simulink model "muscleLegs_task1"  (R2025b)
settings: Solver=ode23t  StartTime=0.0  StopTime=t_end  MaxStep=1e-3  RelTol=1e-4
values from neighbouring files (symbols this model uses):
  c = 0.05    [setup_muscleLegs_nm.m]
  CtrlPar = [tau_H_st; phi_K_tgt_st; P_K_st; D_K_st ... (first row only)    [setup_muscleLegs_ctrl.m]
  eref_se = 0.04    [setup_muscleLegs_nm.m]
  FmaxBFSH = 350    [setup_muscleLegs_nm.m]
  FmaxGLU = 4000    [setup_muscleLegs_nm.m]
  FmaxHFL = 2000    [setup_muscleLegs_nm.m]
  FmaxVAS = 5000    [setup_muscleLegs_nm.m]
  g = 9.81    [setup_muscleLegs_model.m]
  init_stim = 0.01    [setup_muscleLegs_nm.m]
  K = 5    [setup_muscleLegs_nm.m]
  l_shank = l_leg/2    (= 0.49)    [setup_muscleLegs_model.m]
  l_thigh = l_leg/2    (= 0.49)    [setup_muscleLegs_model.m]
  loptBFSH = 0.12    [setup_muscleLegs_nm.m]
  loptGLU = 0.11    [setup_muscleLegs_nm.m]
  loptHFL = 0.11    [setup_muscleLegs_nm.m]
  loptVAS = 0.08    [setup_muscleLegs_nm.m]
  lslackBFSH = 0.10    (= 0.1)    [setup_muscleLegs_nm.m]
  lslackGLU = 0.13    [setup_muscleLegs_nm.m]
  lslackHFL = 0.10    (= 0.1)    [setup_muscleLegs_nm.m]
  lslackVAS = 0.23    [setup_muscleLegs_nm.m]
  m_body = m_total - 2*m_foot    (= 78)    [setup_muscleLegs_model.m]
  m_shank = 4    [setup_muscleLegs_model.m]
  m_thigh = 8    [setup_muscleLegs_model.m]
  N = 12    [cmaes_task1_2_set1.mat]    (also in cmaes_task1_2_set2.mat; cmaes_task2_2_set1.mat = 17; cmaes_task2_2_set2.mat = 17; cmaes_task3_crouch.mat = 17)
  phirefBFSH = 160*pi/180    (= 2.79252680319)    [setup_muscleLegs_nm.m]
  phirefGLU = 60*pi/180    (= 1.0471975512)    [setup_muscleLegs_nm.m]
  phirefHFL = 20*pi/180    (= 0.349065850399)    [setup_muscleLegs_nm.m]
  phirefVAS = 60*pi/180    (= 1.0471975512)    [setup_muscleLegs_nm.m]
  plane_height = 0.1    [setup_muscleLegs_model.m]
  plane_x = 100    [setup_muscleLegs_model.m]
  plane_z = 1    [setup_muscleLegs_model.m]
  r_foot = 0.01    [setup_muscleLegs_model.m]
  rBFSH = 0.04    [setup_muscleLegs_nm.m]
  rGLU = 0.08    [setup_muscleLegs_nm.m]
  rHFL = 0.08    [setup_muscleLegs_nm.m]
  rhoBFSH = 0.7    [setup_muscleLegs_nm.m]
  rhoGLU = 0.5    [setup_muscleLegs_nm.m]
  rhoHFL = 0.5    [setup_muscleLegs_nm.m]
  rhoVAS = 0.6    [setup_muscleLegs_nm.m]
  rVAS = 0.05    [setup_muscleLegs_nm.m]
  tau_act = 0.01    [setup_muscleLegs_nm.m]
  tau_deact = 0.04    [setup_muscleLegs_nm.m]
  vi_Ctrl_st = 1:4    [setup_muscleLegs_ctrl.m]
  vi_Ctrl_sw = 5:12    [setup_muscleLegs_ctrl.m]
  vmaxBFSH = 12    [setup_muscleLegs_nm.m]
  vmaxGLU = 12    [setup_muscleLegs_nm.m]
  vmaxHFL = 12    [setup_muscleLegs_nm.m]
  vmaxVAS = 12    [setup_muscleLegs_nm.m]
  w = 0.56    [setup_muscleLegs_nm.m]
  w_pe = w    (= 0.56)    [setup_muscleLegs_nm.m]
undefined symbols (not defined in the file or in its folder): l1, X, Y, Z
libraries: sm_lib x30, nesl_utility x17, simulink x1
(part 4 of 4)

== system muscleLegs_task1/Muscle Dynamics/MTU7/CE inverse force-velocity relation ==
  note: CE Inverse Force-Velocity Relationship
  Fv[Fmax] : Inport
  1 : Product  Inputs=/*
  Constant{1,3..4,8} (4 alike) : Constant
  Constant2 : Constant  Value=N
  Constant5 : Constant  Value=N
  Curvature : Gain  Gain=K  SaturateOnIntegerOverflow=on  OutDataTypeStr=Inherit: Same as input  ParamDataTypeStr=Inherit: Same as input
  Curvature1 : Gain  Gain=7.56*K  SaturateOnIntegerOverflow=on  OutDataTypeStr=Inherit: Same as input  ParamDataTypeStr=Inherit: Same as input
  Mux : Mux  Inputs=2
  Mux1 : Mux  Inputs=3
  Mux2 : Mux  Inputs=3
  Slope : Gain  Gain=1e-2  SaturateOnIntegerOverflow=on  OutDataTypeStr=Inherit: Same as input  ParamDataTypeStr=Inherit: Same as input
  Sum1 : Sum  Inputs=|++  InputSameDT=on  SaturateOnIntegerOverflow=on  OutDataTypeStr=Inherit: Same as first input
  Sum2 : Sum  InputSameDT=on  SaturateOnIntegerOverflow=on  OutDataTypeStr=Inherit: Same as first input
  Sum3 : Sum  Inputs=++|  InputSameDT=on  SaturateOnIntegerOverflow=on  OutDataTypeStr=Inherit: Same as first input
  Sum4 : Sum  Inputs=|+-  InputSameDT=on  SaturateOnIntegerOverflow=on  OutDataTypeStr=Inherit: Same as first input
  Sum5 : Sum  Inputs=|-+  InputSameDT=on  SaturateOnIntegerOverflow=on  OutDataTypeStr=Inherit: Same as first input
  Sum6 : Sum  Inputs=-+|  InputSameDT=on  SaturateOnIntegerOverflow=on  OutDataTypeStr=Inherit: Same as first input
  Sum7 : Sum  Inputs=|++  InputSameDT=on  SaturateOnIntegerOverflow=on  OutDataTypeStr=Inherit: Same as first input
  Sum8 : Sum  Inputs=+-|  InputSameDT=on  SaturateOnIntegerOverflow=on  OutDataTypeStr=Inherit: Same as first input
  Sum9 : Sum  InputSameDT=on  SaturateOnIntegerOverflow=on  OutDataTypeStr=Inherit: Same as first input
  concentric branch : Fcn  Expr=u(1) * (u(2)<=1)
  excentric branch : Fcn  Expr=u(2) * (u(1)>1)*(u(1)<=u(3))
  excentric overshoot : Fcn  Expr=u(3) * (u(2)>u(1))
  v_concentric : Product  Inputs=*/
  v_excentric <N : Product  Inputs=*/
  v[vmax] : Outport  VectorParamsAs1DForOutWhenUnconnected=off
  wires:
  Curvature/1 -> Sum3/2
  Constant1/1 -> Sum4/2, Sum3/1
  Sum4/1 -> v_concentric/1
  Sum3/1 -> v_concentric/2
  1/1 -> Sum7/1, Curvature1/1
  Constant4/1 -> Sum7/2, Sum8/1
  Curvature1/1 -> Sum8/2
  Sum8/1 -> v_excentric <N/2
  Sum7/1 -> v_excentric <N/1
  v_concentric/1 -> Mux/1
  Fv[Fmax]/1 -> Sum4/1, Curvature/1, Sum6/2, Mux/2, Mux1/1, Mux2/2
  Sum9/1 -> v[vmax]/1
  Sum2/1 -> Sum9/2
  excentric overshoot/1 -> Sum2/2
  Slope/1 -> Sum1/1
  Constant8/1 -> Sum1/2
  Sum6/1 -> 1/2, Slope/1
  Constant2/1 -> Sum6/1, Sum5/2
  Sum5/1 -> 1/1
  Constant3/1 -> Sum5/1
  Mux/1 -> concentric branch/1
  Mux1/1 -> excentric branch/1
  v_excentric <N/1 -> Mux1/2
  Mux2/1 -> excentric overshoot/1
  concentric branch/1 -> Sum9/1
  excentric branch/1 -> Sum2/1
  Constant5/1 -> Mux1/3, Mux2/1
  Sum1/1 -> Mux2/3

== system muscleLegs_task1/Muscle Dynamics/MTU7/PE force-length relation ==
  note: Parallel Elasticity PE
  lce [lopt] : Inport
  Constant3 : Constant
  Math Function2 : Math  Operator=square  SignedPower=on
  Mux : Mux  Inputs=2
  Sum1 : Sum  Inputs=|+-  InputSameDT=on  SaturateOnIntegerOverflow=on  OutDataTypeStr=Inherit: Same as first input
  force above slack length : Fcn  Expr=u(2) * (u(1)>1)
  reference strain [lopt] : Constant  Value=w_pe
  relative strain : Product  Inputs=*/
  fpe [Fmax] : Outport  VectorParamsAs1DForOutWhenUnconnected=off
  wires:
  Mux/1 -> force above slack length/1
  lce [lopt]/1 -> Mux/1, Sum1/1
  Constant3/1 -> Sum1/2
  Sum1/1 -> relative strain/1
  reference strain [lopt]/1 -> relative strain/2
  relative strain/1 -> Math Function2/1
  Math Function2/1 -> Mux/2
  force above slack length/1 -> fpe [Fmax]/1

== system muscleLegs_task1/Muscle Dynamics/MTU7/SE force-length relation ==
  note: SE Force-Length Relationship
  lse [lslack] : Inport
  eref [lslack] : Inport  Port=2
  Constant1 : Constant
  Math Function : Math  Operator=square  SignedPower=on
  Mux : Mux  Inputs=2
  Sum4 : Sum  Inputs=|+-  InputSameDT=on  SaturateOnIntegerOverflow=on  OutDataTypeStr=Inherit: Same as first input
  force above slack length : Fcn  Expr=u(2)*(u(1)>1)
  relative strain : Product  Inputs=*/
  fse [Fmax] : Outport  VectorParamsAs1DForOutWhenUnconnected=off
  wires:
  Mux/1 -> force above slack length/1
  force above slack length/1 -> fse [Fmax]/1
  Math Function/1 -> Mux/2
  lse [lslack]/1 -> Mux/1, Sum4/1
  relative strain/1 -> Math Function/1
  eref [lslack]/1 -> relative strain/2
  Sum4/1 -> relative strain/1
  Constant1/1 -> Sum4/2
